simulink model "robofutebo_socorrol"  (R2015a)
settings: Solver=ode1  StartTime=0.0  StopTime=Tsimu  FixedStep=passo  RelTol=1e-3
values from neighbouring files (symbols this model uses):
  b = 2    [init.m]
  w = 2*pi*(1.5)    (= 9.42477796077)    [init.m]
  x0 = [0 0 (pi/3)*0.8 0 0]'    [init.m]
undefined symbols (not defined in the file or in its folder): xL0
libraries: simulink_extras x1
settings Model: Creator=alessandropeixoto  LastModifiedBy=Jean
settings DataIOCC: SaveFormat=Dataset
settings HardwareCC: ProdBitPerPointer=64  ProdLargestAtomicFloat=Float  ProdIntDivRoundTo=Zero  ProdEndianess=LittleEndian  ProdHWDeviceType=Specified
settings GRTTargetCC: GeneratePreprocessorConditionals=Use local settings

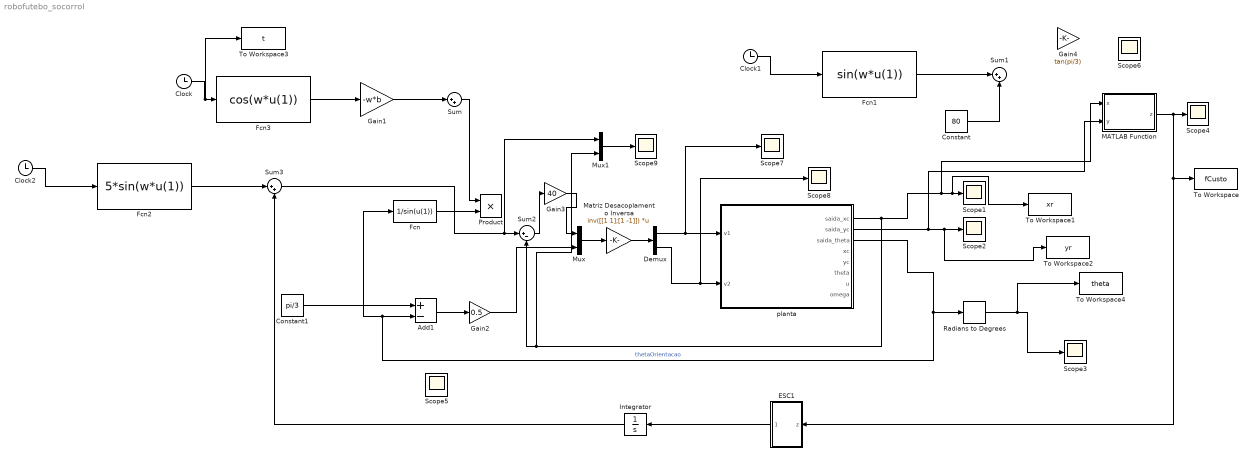
== system robofutebo_socorrol ==
  Add1 : Sum  Inputs=+-
  Clock : Clock
  Clock1 : Clock
  Clock2 : Clock
  Constant : Constant  Value=80
  Constant1 : Constant  Value=pi/3
  Demux : Demux  Outputs=2
  ESC1 : Subsystem
  Fcn : Fcn  Expr=1/sin(u(1))
  Fcn1 : Fcn  Expr=sin(w*u(1))
  Fcn2 : Fcn  Expr=5*sin(w*u(1))
  Fcn3 : Fcn  Expr=cos(w*u(1))
  Gain1 : Gain  Gain=-w*b
  Gain2 : Gain  Gain=0.5
  Gain3 : Gain  Gain=40
  Gain4 : Gain  Gain=tan(pi/3)
  Integrator : Integrator
  MATLAB Function : MATLAB Function  TreatAsAtomicUnit=on
  Matriz Desacoplamento Inversa : Gain  Gain=inv([[1 1];[1 -1]])  Multiplication=Matrix(K*u)
  Mux : Mux  Inputs=2
  Mux1 : Mux  Inputs=2
  Product : Product
  Radians to Degrees : simulink_extras/Transformations/Radians to Degrees
  Scope{1..9} (9 alike) : Scope
      Scope1 settings: YMin=65  YMax=72.5
      Scope2 settings: YMin=41.95  YMax=42.375  SaveName=ScopeData2
      Scope3 settings: YMin=49  YMax=64  SaveName=ScopeData3
      Scope4 settings: TimeRange=80  YMin=-51.25  YMax=-50.5
      Scope5 settings: YMin=-12.75  YMax=-9  SaveName=ScopeData4
      Scope6 settings: YMin=-40000  YMax=-7500  SaveName=ScopeData9
      Scope7 settings: YMin=-600  YMax=700  SaveName=ScopeData10
      Scope8 settings: YMin=57  YMax=63  SaveName=ScopeData11
      Scope9 settings: YMin=55  YMax=120  SaveName=ScopeData14
  Sum : Sum  Inputs=|++
  Sum1 : Sum  Inputs=|++
  Sum2 : Sum  Inputs=|+-
  Sum3 : Sum  Inputs=|++
  To Workspace : ToWorkspace  VariableName=fCusto  SampleTime=-1
  To Workspace1 : ToWorkspace  VariableName=xr  SampleTime=-1
  To Workspace2 : ToWorkspace  VariableName=yr  SampleTime=-1
  To Workspace3 : ToWorkspace  VariableName=t  SampleTime=-1
  To Workspace4 : ToWorkspace  VariableName=theta  SampleTime=-1
  planta : Subsystem
  wires:
  Add1/1 -> Gain2/1
  planta/1(saida_xc) -> MATLAB Function/1(x), To Workspace1/1, Scope1/1, Mux1/2, Sum2/2
  planta/2(saida_yc) -> MATLAB Function/2(y), To Workspace2/1, Scope2/1
  planta/3(saida_theta) -> Fcn/1, Add1/2, Radians to Degrees/1  "thetaOrientacao"
  Matriz Desacoplamento Inversa/1 -> Demux/1
  Demux/1 -> Scope7/1, planta/1(v1)
  Demux/2 -> Scope8/1, planta/2(v2)
  Gain2/1 -> Mux/2
  Constant1/1 -> Add1/1
  Fcn/1 -> Product/2
  Clock/1 -> To Workspace3/1, Fcn3/1
  Fcn3/1 -> Gain1/1
  Gain1/1 -> Sum/1
  Sum/1 -> Product/1
  ESC1/1(uesc) -> Integrator/1
  MATLAB Function/1(z) -> To Workspace/1, ESC1/1(z), Scope4/1
  Clock1/1 -> Fcn1/1
  Fcn1/1 -> Sum1/1
  Constant/1 -> Sum1/2
  Sum2/1 -> Gain3/1
  Gain3/1 -> Mux/1
  Mux/1 -> Matriz Desacoplamento Inversa/1
  Integrator/1 -> Sum3/2
  Clock2/1 -> Fcn2/1
  Fcn2/1 -> Sum3/1
  Sum3/1 -> Mux1/1, Sum2/1
  Mux1/1 -> Scope9/1
  Radians to Degrees/1 -> To Workspace4/1, Scope3/1

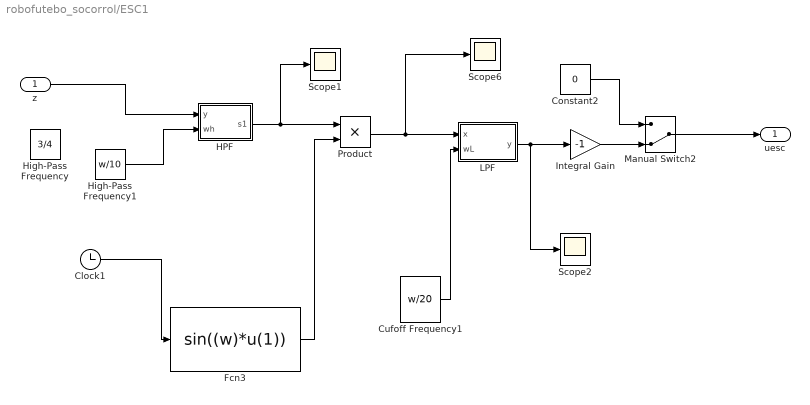
== system robofutebo_socorrol/ESC1 ==
  z : Inport
  Clock1 : Clock
  Constant2 : Constant  Value=0
  Cufoff Frequency1 : Constant  Value=w/20  SampleTime=Inf
  Fcn3 : Fcn  Expr=sin((w)*u(1))
  HPF : Subsystem
  High-Pass Frequency : Constant  Value=3/4  SampleTime=Inf
  High-Pass Frequency1 : Constant  Value=w/10  SampleTime=Inf
  Integral Gain : Gain  Gain=-1
  LPF : Subsystem
  Manual Switch2 : ManualSwitch  CurrentSetting=0
  Product : Product
  Scope1 : Scope
      settings: YMin=0.5  YMax=12  SaveName=ScopeData6
  Scope2 : Scope
      settings: YMin=-1  YMax=1  SaveName=ScopeData8
  Scope6 : Scope
      settings: YMin=-0.2  YMax=0.25  SaveName=ScopeData7
  uesc : Outport
  wires:
  Constant2/1 -> Manual Switch2/1
  z/1 -> HPF/1(y)
  Clock1/1 -> Fcn3/1
  HPF/1(s1) -> Product/1, Scope1/1
  LPF/1(y) -> Integral Gain/1, Scope2/1
  Integral Gain/1 -> Manual Switch2/2
  Manual Switch2/1 -> uesc/1
  Product/1 -> Scope6/1, LPF/1(x)
  High-Pass Frequency1/1 -> HPF/2(wh)
  Fcn3/1 -> Product/2
  Cufoff Frequency1/1 -> LPF/2(wL)

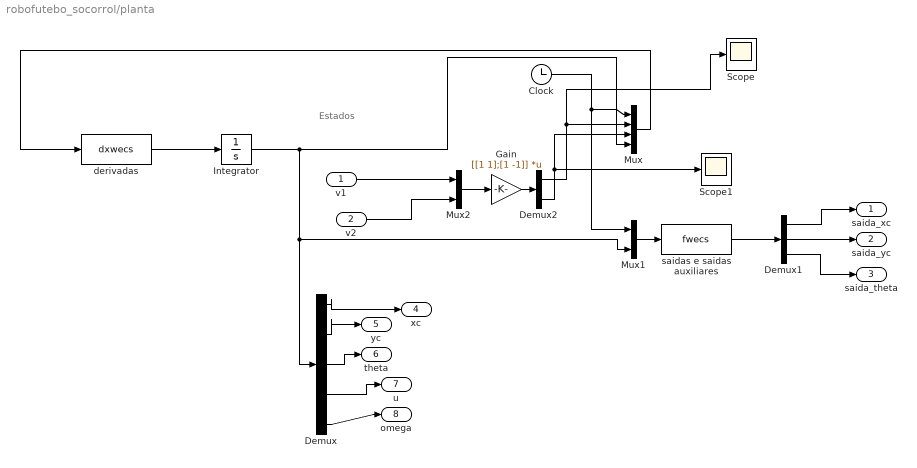
== system robofutebo_socorrol/planta ==
  note: Estados
  v1 : Inport
  v2 : Inport  Port=2
  Clock : Clock
  Demux : Demux  Outputs=5
  Demux1 : Demux  Outputs=3
  Demux2 : Demux  Outputs=2
  Gain : Gain  Gain=[[1 1];[1 -1]]  Multiplication=Matrix(K*u)
  Integrator : Integrator  InitialCondition=x0
  Mux : Mux
  Mux1 : Mux  Inputs=2
  Mux2 : Mux  Inputs=2
  Scope : Scope
      settings: SaveName=ScopeData12
  Scope1 : Scope
      settings: SaveName=ScopeData13
  derivadas : MATLABFcn  MATLABFcn=dxwecs
  saidas e saidas auxiliares : MATLABFcn  MATLABFcn=fwecs
  saida_xc : Outport
  saida_yc : Outport  Port=2
  saida_theta : Outport  Port=3
  xc : Outport  Port=4
  yc : Outport  Port=5
  theta : Outport  Port=6
  u : Outport  Port=7
  omega : Outport  Port=8
  wires:
  Clock/1 -> Mux1/1, Mux/1
  Mux/1 -> derivadas/1
  Integrator/1 -> Mux/4, Demux/1, Mux1/2
  Demux/4 -> u/1
  Demux/5 -> omega/1
  derivadas/1 -> Integrator/1
  Mux1/1 -> saidas e saidas auxiliares/1
  saidas e saidas auxiliares/1 -> Demux1/1
  Demux1/1 -> saida_xc/1
  Demux1/2 -> saida_yc/1
  Demux/1 -> xc/1
  Demux/2 -> yc/1
  Demux/3 -> theta/1
  Demux1/3 -> saida_theta/1
  v1/1 -> Mux2/1
  v2/1 -> Mux2/2
  Mux2/1 -> Gain/1
  Gain/1 -> Demux2/1
  Demux2/1 -> Scope/1, Mux/2
  Demux2/2 -> Scope1/1, Mux/3

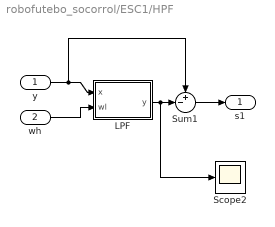
== system robofutebo_socorrol/ESC1/HPF ==
  y : Inport
  wh : Inport  Port=2
  LPF : Subsystem
  Scope2 : Scope
      settings: YMin=0.6  YMax=1.125  SaveName=ScopeData5
  Sum1 : Sum  Inputs=+-|
  s1 : Outport
  wires:
  LPF/1(y) -> Sum1/2, Scope2/1
  wh/1 -> LPF/2(wl)
  Sum1/1 -> s1/1
  y/1 -> Sum1/1, LPF/1(x)

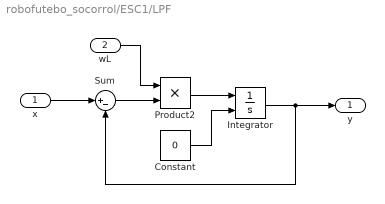
== system robofutebo_socorrol/ESC1/LPF ==
  x : Inport
  wL : Inport  Port=2
  Constant : Constant  Value=0
  Integrator : Integrator  InitialConditionSource=external  InitialCondition=xL0
  Product2 : Product
  Sum : Sum  Inputs=|+-
  y : Outport
  wires:
  Constant/1 -> Integrator/2
  x/1 -> Sum/1
  Sum/1 -> Product2/2
  Product2/1 -> Integrator/1
  Integrator/1 -> y/1, Sum/2
  wL/1 -> Product2/1

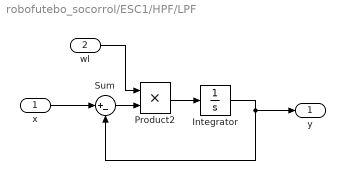
== system robofutebo_socorrol/ESC1/HPF/LPF ==
  x : Inport
  wl : Inport  Port=2
  Integrator : Integrator
  Product2 : Product
  Sum : Sum  Inputs=|+-
  y : Outport
  wires:
  wl/1 -> Product2/1
  Integrator/1 -> y/1, Sum/2
  Product2/1 -> Integrator/1
  Sum/1 -> Product2/2
  x/1 -> Sum/1

== matlab function robofutebo_socorrol/MATLAB Function ==
  data: x input; y input; z output
function z = fcn(x,y)
%#codegen
%vetorDistancia = sqrt(u1^2+u2^2);
%exp = -((vetorDistancia-80)^2)/10+10;
exp = (-((x-50)^2+(y-86.60)^2))/10+10;

z = exp;
